simulink model "stanley01"  (R2022a)
settings: Solver=VariableStepAuto  StartTime=0.0  StopTime=70  RelTol=1e-3
values from neighbouring files (symbols this model uses):
  cx = 0:0.1:120    [stanley_ref_01.m]
  cy = dy1/2.*(1+tanh(z1))-dy2/2.*(1+tanh(z2))    [stanley_ref_01.m]
  r_yaw = atan2(dif_yyyy , dif_xxxx)    [stanley_ref_01.m]
libraries: Solver_SF x1, simulink x1
settings Model: Creator=wenju  LastModifiedBy=wenju

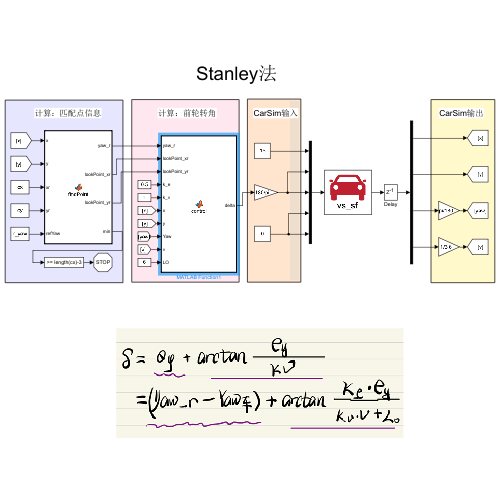
[thumbnail: Simulink's stored preview of the top-level diagram]
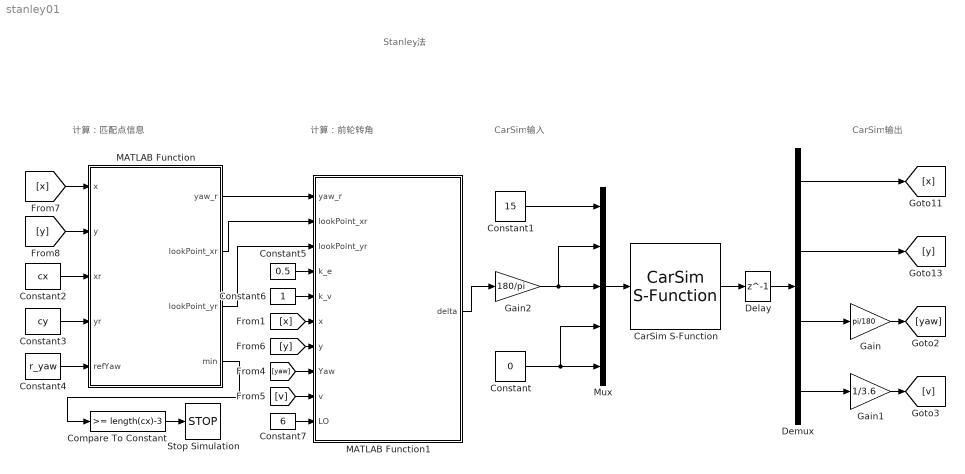
== system stanley01 ==
  note: Stanley法
  note: CarSim输入
  note: CarSim输出
  note: 计算：前轮转角
  note: 计算：匹配点信息
  CarSim S-Function : Solver_SF/CarSim S-Function  Priority=1  SIMFILE=simfile.sim  Run_RTs=off  vs_state_ind=Run  StopMode_ind=Vehicle Model
  Compare To Constant : simulink/Logic and Bit Operations/Compare To Constant  relop=>=  const=length(cx)-3  OutDataTypeStr=boolean
  Constant : Constant  Value=0
  Constant1 : Constant  Value=15
  Constant2 : Constant  Value=cx
  Constant3 : Constant  Value=cy
  Constant4 : Constant  Value=r_yaw
  Constant5 : Constant  Value=0.5
  Constant6 : Constant
  Constant7 : Constant  Value=6
  Delay : Delay  DelayLength=1  InitialCondition=0  UseCircularBuffer=on
  Demux : Demux
  Gain : Gain  Gain=pi/180
  Gain1 : Gain  Gain=1/3.6
  Gain2 : Gain  Gain=180/pi
  MATLAB Function : MATLAB Function  TreatAsAtomicUnit=on
  MATLAB Function1 : MATLAB Function  TreatAsAtomicUnit=on
  Mux : Mux  Inputs=5
  Stop Simulation : Stop
  wires:
  Mux/1 -> CarSim S-Function/1
  CarSim S-Function/1 -> Delay/1
  Delay/1 -> Demux/1
  Demux/1 -> [x]
  Demux/3 -> Gain/1
  Gain/1 -> [yaw]
  Demux/4 -> Gain1/1
  Gain1/1 -> [v]
  Constant/1 -> Mux/4, Mux/5
  Gain2/1 -> Mux/2, Mux/3
  Constant2/1 -> MATLAB Function/3(xr)
  Constant3/1 -> MATLAB Function/4(yr)
  Constant4/1 -> MATLAB Function/5(refYaw)
  MATLAB Function/3(lookPoint_yr) -> MATLAB Function1/3(lookPoint_yr)
  MATLAB Function/2(lookPoint_xr) -> MATLAB Function1/2(lookPoint_xr)
  MATLAB Function/1(yaw_r) -> MATLAB Function1/1(yaw_r)
  [yaw] -> MATLAB Function1/8(Yaw)
  [v] -> MATLAB Function1/9(v)
  Constant5/1 -> MATLAB Function1/4(k_e)
  Constant6/1 -> MATLAB Function1/5(k_v)
  MATLAB Function/4(min) -> Compare To Constant/1
  Compare To Constant/1 -> Stop Simulation/1
  MATLAB Function1/1(delta) -> Gain2/1
  Demux/2 -> [y]
  [x] -> MATLAB Function1/6(x)
  [y] -> MATLAB Function1/7(y)
  Constant7/1 -> MATLAB Function1/10(LO)
  [x] -> MATLAB Function/1(x)
  [y] -> MATLAB Function/2(y)
  Constant1/1 -> Mux/1

== matlab function stanley01/MATLAB Function1 ==
  data: yaw_r input; lookPoint_xr input; lookPoint_yr input; k_e input; k_v input; x input; delta output; y input; Yaw input; v input; LO input
%****************************获得控制量：前轮转向*************************

function delta = control(yaw_r,lookPoint_xr,lookPoint_yr,k_e,k_v,x,y,Yaw,v,LO)
%*******************CarSim转角向左为正*************************************

%横向误差：两点距离
e_y=sqrt((x-lookPoint_xr)^2+(y-lookPoint_yr)^2);

%判断转向：转换到车辆坐标系下的 纵坐标 正负，小于0，需要向右拐，让其为负值
dx=x-lookPoint_xr;
dy=y-lookPoint_yr;
L_R = dy*cos(Yaw) - dx*sin(Yaw);

if L_R < 0
   e_y = -e_y;     
end

%横向误差产生的控制量
ey_yaw=atan2(-k_e*e_y,k_v*v+LO);
%对控制量角度进行限制，使其始终在  -pi到pi之间
if ey_yaw > pi
    ey_yaw = ey_yaw - 2*pi;
end
if ey_yaw < -pi
    ey_yaw = ey_yaw + 2*pi;
end

%转角误差：CarSim转角向左为正，自动满足
ehead_yaw=yaw_r-Yaw;
%对控制量角度进行限制，使其始终在  -pi到pi之间
if ehead_yaw > pi
    ehead_yaw = ehead_yaw - 2*pi;
end
if ehead_yaw < -pi
    ehead_yaw = ehead_yaw + 2*pi;
end


%最两部分组成终前轮转角：
delta = ehead_yaw+ey_yaw;
%对最终控制量进行限制，这里假设车辆  向左最多只能转pi/6，向右最多只能转pi/6
if delta > pi/6
    delta = pi/6;
end
if delta < -pi/6
    delta = -pi/6;
end

end

== matlab function stanley01/MATLAB Function ==
  data: yaw_r output; lookPoint_xr output; lookPoint_yr output; x input; min output; y input; xr input; yr input; refYaw input
% 首先在参考轨迹上搜索离当前车辆位置最近的点
function [yaw_r,lookPoint_xr, lookPoint_yr,min] = findPoint(x,y, xr,yr,refYaw)

% 找到距离当前位置最近的一个参考轨迹点的序号
n=length(xr);
d_min=(x-xr(1))^2+(y-yr(1))^2;
min=1;
for i = 1:n
    d = (x-xr(i))^2+(y-yr(i))^2; 
    if d<d_min
        d_min=d;
        min=i;
    end
end

%通过轨迹点序号得出相关轨迹x,y位置信息与切线夹角
lookPoint_xr = xr(min);
lookPoint_yr = yr(min);
yaw_r=refYaw(min);

end
